simulink model "CPS_Eva"  (R2022b)
settings: Solver=ode5  StartTime=0.0  StopTime=duration_sim  RelTol=1e-3
model workspace (MAT data in the model file):
  mass_of_cylinder = 0.306
values from neighbouring files (symbols this model uses):
  c = 2*dampratio*sqrt(k*M)    [CPS_sims_and_analysis.m]    (also in command_limits_check.m; ringdown-circcyl-M10-d0_001-F1-workspace.mat = 0.125663706144; setup_CPS_parameters.m)
  Gromit_Cal_tranp = [-0.02196001634 0.004190267995 -0.186118155718 -17.4835109711 1.2242256403 16.6441669464 0.965337395668 19.7935447693 -0.233169600368 -10.1337041855 -0.765193104744 -9.66913127899 ... (36 elements, 6x6)]    [ringdown-circcyl-M10-d0_001-F1-workspace.mat]    (also in setup_CPS_parameters.m = Gromit_Cal')
  k = (2*pi*f_nat)^2*M    (= 394.784176044)    [CPS_sims_and_analysis.m]    (also in command_limits_check.m = 98.6960440109; ringdown-circcyl-M10-d0_001-F1-workspace.mat; setup_CPS_parameters.m)
  M = 10    [CPS_sims_and_analysis.m]    (also in command_limits_check.m; ringdown-circcyl-M10-d0_001-F1-workspace.mat; setup_CPS_parameters.m)
  start_position_cm = 10    [command_limits_check.m]    (also in ringdown-circcyl-M10-d0_001-F1-workspace.mat = 0.0117475; setup_CPS_parameters.m = 0)
  T = 0.0002    [ringdown-circcyl-M10-d0_001-F1-workspace.mat]    (also in setup_CPS_parameters.m)
undefined symbols (not defined in the file or in its folder): DiscIntNeverNeededParam, Fx, Fy, Fy_plus_ma_filtered, ma, National_Instruments, PCIe, sigbuilder_block, torque_z
libraries: sldrtlib x5, dsparch4 x1
settings Model: SimulationMode=external  ExtModeTrigDuration=1000000  Creator=eericks1  LastModifiedBy=eericks1
settings DataIOCC: ReturnWorkspaceOutputs=off
settings DebuggingCC: ReadBeforeWriteMsg=DisableAll  WriteAfterWriteMsg=DisableAll  WriteAfterReadMsg=DisableAll  MultiTaskDSMMsg=none
settings HardwareCC: ProdBitPerLong=64  ProdHWDeviceType=Intel->x86-64 (Linux 64)
settings ModelReferenceCC: UpdateModelReferenceTargets=IfOutOfDate
settings SFSimCC: SFSimEcho=off
settings RTWCC: Description=Simulink Desktop Real-Time  SystemTargetFile=sldrt.tlc  TemplateMakefile=sldrt.tmf  RTWCompilerOptimization=on
settings CodeAppCC: MaxIdLength=95
settings SimulinkDesktopRealTimeCC: TargetLibSuffix=_sldrt.a  TargetPreCompLibLocation=C:\Program Files\MATLAB\R2022b\toolbox\sldrt\lib\win64

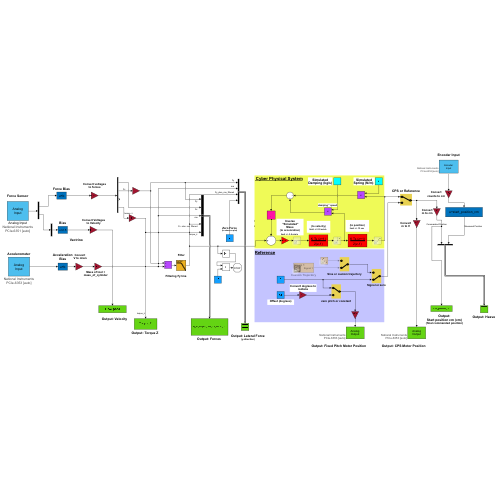
[thumbnail: Simulink's stored preview of the top-level diagram]
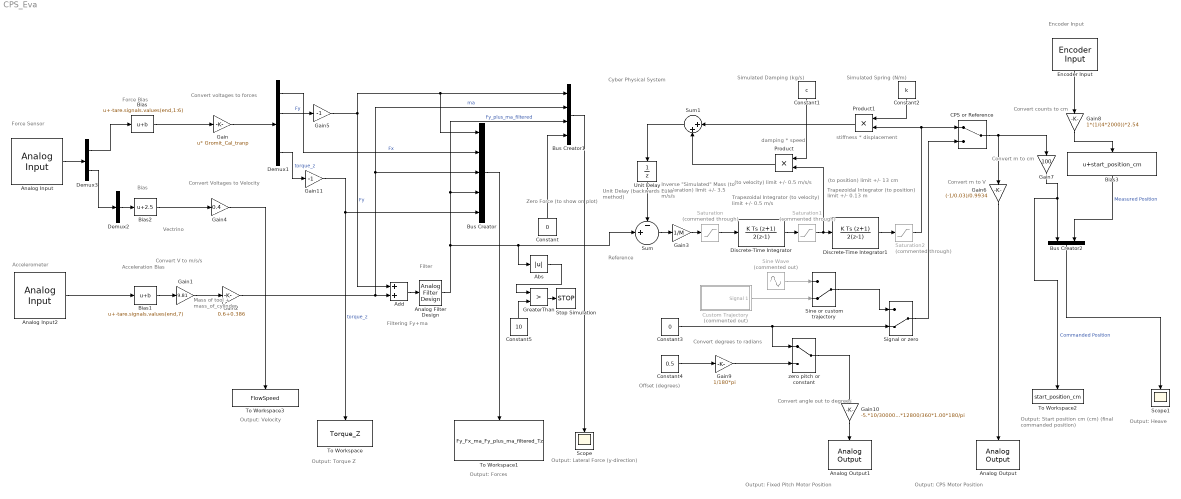
== system CPS_Eva ==
  note: Convert voltages to forces
  note: Simulated
      | Spring (N/m)
  note: Mass of tool + mass_of_cylinder
  note: Simulated
      | Damping (kg/s)
  note: Offset (degrees)
  note: Output: Forces
  note: Inverse
      | "Simulated"
      | Mass
      | (to acceleration)
      | limit +/- 3.5 m/s/s
  note: Output: Lateral Force
      | (y-direction)
  note: Convert Voltages to Velocity
  note: damping * speed
  note: Convert
      | counts to cm
  note: Cyber Physical System
  note: Zero Force
      | (to show on plot)
  note: Output: Velocity
  note: Unit Delay
      | (backwards
      | Euler method)
  note: Convert
      | m to cm
  note: Output: Heave
  note: Acceleration
      | Bias
  note: Convert degrees to radians
  note: Reference
  note: Trapezoidal Integrator
      | (to position)
      | limit +/- 0.13 m
  note: Bias
  note: Output: Torque Z
  note: Convert
      | V to m/s/s
  note: stiffness * displacement
  note: Force Sensor
  note: Convert
      | m to V
  note: Trapezoidal Integrator
      | (to velocity)
      | limit +/- 0.5 m/s
  note: Force Bias
  note: Encoder Input
  note: Convert angle out to degrees
  note: Accelerometer
  note: Output: Fixed Pitch Motor Position
  note: Filter
  note: Output: CPS Motor Position
  note: Output:
      | Start position cm (cm)
      | (final commanded position)
  note: Filtering Fy+ma
  note: Vectrino
  note: (to velocity)
      | limit +/- 0.5 m/s/s
  note: (to position)
      | limit +/- 13 cm
  Abs : Abs  SaturateOnIntegerOverflow=off
  Add : Sum
  Analog Filter Design : dsparch4/Analog Filter Design  method=Butterworth  filttype=Lowpass  N=4  Wlo=2*3.14*10  Whi=80  Rp=2  Rs=40
  Analog Input : sldrtlib/Analog Input  SampleTime=T  MaxMissedTicks=10  ShowMissedTicks=off  YieldWhenWaiting=off  DrvName=National_Instruments/PCIe-6351  DrvAddress=4294967295  DrvOptions=[0 0 0 0 0 0 0]  Channels=[1:10]  RangeMode=1  VoltRange=1  DataType=1
      settings: AttributesFormatString=National Instruments\nPCIe-6351 [auto]
  Analog Input2 : sldrtlib/Analog Input  SampleTime=T  MaxMissedTicks=10  ShowMissedTicks=off  YieldWhenWaiting=off  DrvName=National_Instruments/PCIe-6353  DrvAddress=4294967295  DrvOptions=[0 0 0 2 2 2 2]  Channels=[25]  RangeMode=1  VoltRange=1  DataType=1
      settings: AttributesFormatString=National Instruments\nPCIe-6353 [auto]
  Analog Output : sldrtlib/Analog Output  SampleTime=T  MaxMissedTicks=10  ShowMissedTicks=off  YieldWhenWaiting=off  DrvName=National_Instruments/PCIe-6353  DrvAddress=4294967295  DrvOptions=[0 0 0 2 2 2 2]  Channels=[4]  RangeMode=1  VoltRange=1  InitialValue=[]  FinalValue=[]
      settings: AttributesFormatString=National Instruments\nPCIe-6353 [auto]
  Analog Output1 : sldrtlib/Analog Output  SampleTime=T  MaxMissedTicks=10  ShowMissedTicks=off  YieldWhenWaiting=off  DrvName=National_Instruments/PCIe-6353  DrvAddress=4294967295  DrvOptions=[0 0 0 2 2 2 2]  Channels=[3]  RangeMode=1  VoltRange=1  InitialValue=[]  FinalValue=[]
      settings: AttributesFormatString=National Instruments\nPCIe-6353 [auto]
  Bias : Bias  Bias=-tare.signals.values(end,1:6)  SaturateOnIntegerOverflow=off
  Bias1 : Bias  Bias=-tare.signals.values(end,7)  SaturateOnIntegerOverflow=off
  Bias2 : Bias  Bias=2.5  SaturateOnIntegerOverflow=off
  Bias3 : Bias  Bias=start_position_cm  SaturateOnIntegerOverflow=off
  Bus Creator : BusCreator  Inputs=Fy,Fx,ma,Fy_plus_ma_filtered,torque_z
  Bus Creator1 : BusCreator  Inputs=4
  Bus Creator2 : BusCreator  Inputs=2
  CPS or Reference : ManualSwitch
  Constant : Constant  Value=0  SampleTime=T
  Constant1 : Constant  Value=c  SampleTime=T
  Constant2 : Constant  Value=k  SampleTime=T
  Constant3 : Constant  Value=0  SampleTime=T
  Constant4 : Constant  Value=0.5  SampleTime=T
  Constant5 : Constant  Value=10  SampleTime=T
  Custom Trajectory : Subsystem  Tag=STV Subsys  Commented=on  LoadFcn=sigbuilder_block('load');  StartFcn=sigbuilder_block('start');  StopFcn=sigbuilder_block('stop');  ClipboardFcn=sigbuilder_block('clipboard');  mask(Sigbuilder block){tuvar=[0:10]}
      mask help: Simulink:masks:SigbuilderBlock_MD
      mask init:
      | if ~strcmp(get_param(bdroot(gcbh),'SimulationStatus'),'stopped') tuvar = sigbuilder_block('maskInit'); end
      settings: CopyFcn=sigbuilder_block('copy');  DeleteFcn=sigbuilder_block('delete');  ModelCloseFcn=sigbuilder_block('modelClose');  PreSaveFcn=sigbuilder_block('preSave');  PauseFcn=sigbuilder_block('pause');  ContinueFcn=sigbuilder_block('continue');  NameChangeFcn=sigbuilder_block('namechange');  OpenFcn=sigbuilder_block('open',[135.75 180.75 550.5 399.75 ]);  CloseFcn=sigbuilder_block('close');
      mask Display: plot(0, 0, 100, 100,[2, 2, 32, 32, 2], [68, 8, 8, 68, 68],[32, 2], [38, 38], [32, 19, 2],[53, 60, 44], [32, 17, 17, 2],[16, 16, 31, 31]);txt = getActiveGroup(gcbh);text(2, 100, txt,'verticalAlignment', 'top');
  Demux1 : Demux  Outputs=[1 1 3 1]
  Demux2 : Demux  Outputs=[4]
  Demux3 : Demux  Outputs=[6 4]
  Discrete-Time Integrator : DiscreteIntegrator  IntegratorMethod=Integration: Trapezoidal  SampleTime=-1  UpperSaturationLimit=0.5  LowerSaturationLimit=-0.5  ICPrevOutput=DiscIntNeverNeededParam  ICPrevScaledInput=DiscIntNeverNeededParam
  Discrete-Time Integrator1 : DiscreteIntegrator  IntegratorMethod=Integration: Trapezoidal  InitialCondition=start_position_cm/100  SampleTime=-1  UpperSaturationLimit=.13  LowerSaturationLimit=-.13  ICPrevOutput=DiscIntNeverNeededParam  ICPrevScaledInput=DiscIntNeverNeededParam
  Encoder Input : sldrtlib/Encoder Input  SampleTime=T  MaxMissedTicks=10  ShowMissedTicks=off  YieldWhenWaiting=off  DrvName=National_Instruments/PCIe-6353  DrvAddress=4294967295  DrvOptions=[0 0 0 2 2 2 2]  Channels=[1]  QuadMode=3  IndexPulse=1  InputFilter=Inf  DataType=1
      settings: AttributesFormatString=National Instruments\nPCIe-6353 [auto]
  Gain : Gain  Gain=Gromit_Cal_tranp  Multiplication=Matrix(u*K)
  Gain1 : Gain  Gain=9.81
  Gain10 : Gain  Gain=-5.*10/30000*12800/360*1.00*180/pi
  Gain11 : Gain  Gain=-1
  Gain2 : Gain  Gain=0.6+0.386
  Gain3 : Gain  Gain=1/M
  Gain4 : Gain  Gain=0.4
  Gain5 : Gain  Gain=-1
  Gain6 : Gain  Gain=(-1/0.03)/0.9934
  Gain7 : Gain  Gain=100
  Gain8 : Gain  Gain=1*(1/(4*2000))*2.54
  Gain9 : Gain  Gain=1/180*pi
  GreaterThan : RelationalOperator  Operator=>  OutDataTypeStr=boolean  RndMeth=Simplest  InputSameDT=off
  Product : Product
  Product1 : Product
  Saturation : Saturate  Commented=through  UpperLimit=3.5  LowerLimit=-3.5
  Saturation1 : Saturate  Commented=through
  Saturation2 : Saturate  Commented=through  UpperLimit=0.13  LowerLimit=-0.13
  Scope : Scope
  Scope1 : Scope
  Signal or zero : ManualSwitch  CurrentSetting=0
  Sine Wave : Sin  Commented=on  Amplitude=0.05  Frequency=2*3.14*1  SampleTime=0
  Sine or custom trajectory : ManualSwitch  CurrentSetting=0
  Stop Simulation : Stop
  Sum : Sum  Inputs=-+|
  Sum1 : Sum  Inputs=|++
  To Workspace : ToWorkspace  VariableName=Torque_Z  SaveFormat=Structure With Time  SampleTime=-1
  To Workspace1 : ToWorkspace  VariableName=Fy_Fx_ma_Fy_plus_ma_filtered_Tz  SampleTime=-1
      settings: Save2DSignal=2-D array (concatenate along first dimension)
  To Workspace2 : ToWorkspace  VariableName=start_position_cm  SampleTime=-1
      settings: MaxDataPoints=1  Save2DSignal=2-D array (concatenate along first dimension)
  To Workspace3 : ToWorkspace  VariableName=FlowSpeed  SaveFormat=Structure With Time  SampleTime=-1
  Unit Delay : UnitDelay  InitialCondition=start_position_cm*k/100  SampleTime=-1  HasFrameUpgradeWarning=on
  zero pitch or constant : ManualSwitch
  wires:
  Demux3/2 -> Demux2/1
  Saturation1/1 -> Product/2, Discrete-Time Integrator1/1
  Constant2/1 -> Product1/1
  Analog Input2/1 -> Bias1/1
  Demux3/1 -> Bias/1
  Encoder Input/1 -> Gain8/1
  Bus Creator1/1 -> Scope/1
  Gain8/1 -> Bias3/1
  zero pitch or constant/1 -> Gain10/1
  Demux1/1 -> Bus Creator/2  "Fx"
  Gain10/1 -> Analog Output1/1
  Analog Input/1 -> Demux3/1
  Constant4/1 -> Gain9/1
  Analog Filter Design/1 -> Bus Creator1/3, Bus Creator/4, Abs/1, Sum/2  "Fy_plus_ma_filtered"
  Saturation/1 -> Discrete-Time Integrator/1
  Gain5/1 -> Add/1, Bus Creator/1, Bus Creator1/1  "Fy"
  Gain4/1 -> To Workspace3/1
  Product1/1 -> Sum1/1
  Constant/1 -> Bus Creator1/4
  Add/1 -> Analog Filter Design/1
  Sum1/1 -> Unit Delay/1
  CPS or Reference/1 -> Gain7/1, Gain6/1
  Demux1/2 -> Gain5/1  "Fy"
  Sum/1 -> Gain3/1
  Bias1/1 -> Gain1/1
  Constant3/1 -> Signal or zero/2, zero pitch or constant/1
  Sine or custom trajectory/1 -> Signal or zero/1
  Gain11/1 -> Bus Creator/5, To Workspace/1  "torque_z"
  Gain9/1 -> zero pitch or constant/2
  Bias3/1 -> Bus Creator2/2  "Measured Position"
  Signal or zero/1 -> CPS or Reference/2
  Gain2/1 -> Bus Creator/3, Bus Creator1/2, Add/2  "ma"
  Gain1/1 -> Gain2/1
  Sine Wave/1 -> Sine or custom trajectory/1
  Gain7/1 -> To Workspace2/1, Bus Creator2/1  "Commanded Position"
  Unit Delay/1 -> Sum/1
  Discrete-Time Integrator1/1 -> Saturation2/1
  Bus Creator2/1 -> Scope1/1
  Constant1/1 -> Product/1
  Saturation2/1 -> Product1/2, CPS or Reference/1
  Demux2/1 -> Bias2/1
  Discrete-Time Integrator/1 -> Saturation1/1
  Gain/1 -> Demux1/1
  Bus Creator/1 -> To Workspace1/1
  Bias/1 -> Gain/1
  Demux1/4 -> Gain11/1  "torque_z"
  Gain6/1 -> Analog Output/1
  Gain3/1 -> Saturation/1
  Custom Trajectory/1(Signal 1) -> Sine or custom trajectory/2
  Bias2/1 -> Gain4/1
  Product/1 -> Sum1/2
  GreaterThan/1 -> Stop Simulation/1
  Constant5/1 -> GreaterThan/2
  Abs/1 -> GreaterThan/1

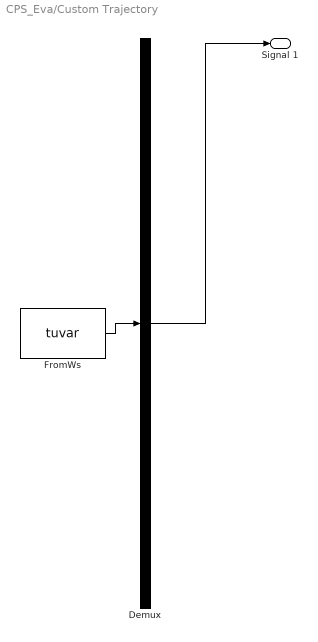
== system CPS_Eva/Custom Trajectory ==
  Demux : Demux  Tag=STV Demux  Outputs=1
      settings: DisplayOption=none
  FromWs : FromWorkspace  Tag=STV FromWs  VariableName=tuvar
      SigBuilderData=|
      | common.afterFinalStr = 'Extrapolate'
      | common.sampleTime = 0
      | dataSet.timeRange = [0 10]
      | dataSet.name = 'Group 1'
      | sbobj.Groups.Name = 'Group 1'
      | sbobj.Groups.Signals.Name = 'Signal 1'
      | sbobj.Groups.Signals.XData = [0 0.0005 0.001 0.0015 0.002 0.0025 0.003 0.0035 0.004 0.0045 0.005 0.0055 ... (1762 elements, 1x1762)]
      | sbobj.Groups.Signals.YData = [0 5.08130081301e-07 2.0325203252e-06 4.57317073171e-06 8.13008130081e-06 1.27032520325e-05 1.82926829268e-05 2.48983739837e-05 3.25203252033e-05 4.11585365854e-05 5.08130081301e-05 6.14837398374e-05 ... (1762 elements, 1x1762)]
  Signal 1 : Outport  Tag=STV Outport
  wires:
  Demux/1 -> Signal 1/1
  FromWs/1 -> Demux/1
